simulink model "SimpleECU"  (R2024b)
settings: configuration reference "EngFixed10ms" (kept outside this file)
undefined symbols (not defined in the file): CtrlEcuRevLim
settings Model: DataDictionary=VirtualDynoTemplate.sldd  ModifiedByFormat=The MathWorks, Inc.  Creator=The MathWorks, Inc.  LastModifiedBy=The MathWorks, Inc.
settings ConfigSetRef: SourceName=EngFixed10ms

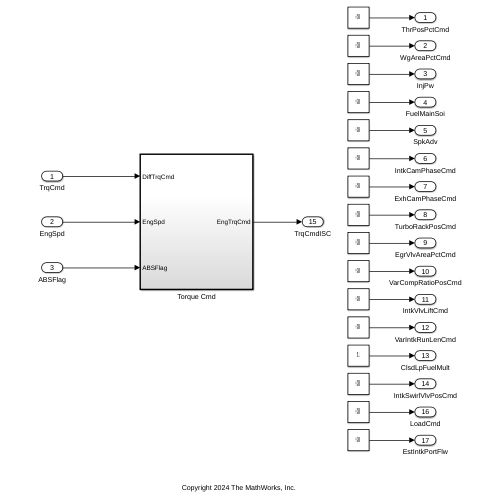
[thumbnail: Simulink's stored preview of the top-level diagram]
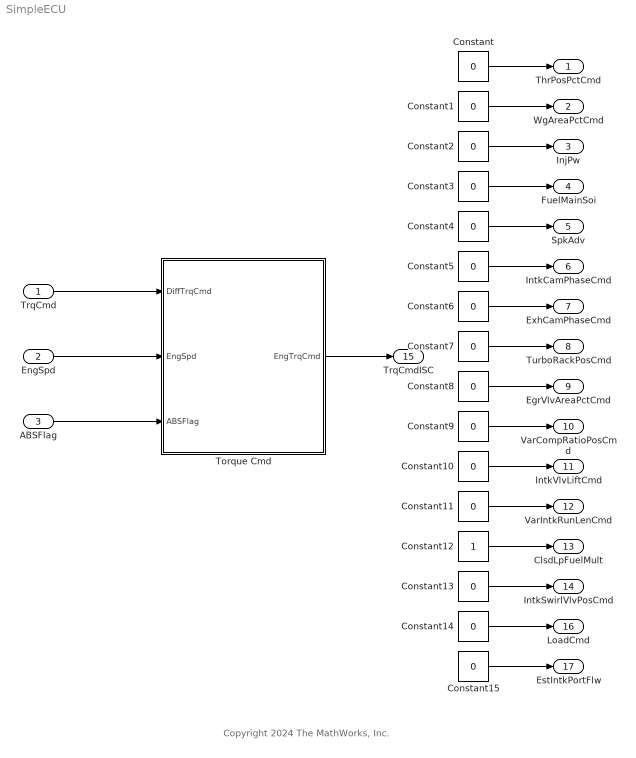
== system SimpleECU ==
  note: Copyright 2024 The MathWorks, Inc.
  TrqCmd : Inport
  EngSpd : Inport  Port=2
  ABSFlag : Inport  Port=3  OutDataTypeStr=boolean
  Constant{,1..11,13..15} (15 alike) : Constant  Value=0  SampleTime=-1
  Constant12 : Constant  SampleTime=-1
  Torque Cmd : Subsystem  TreatAsAtomicUnit=on  SystemSampleTime=.01
  ThrPosPctCmd : Outport  VectorParamsAs1DForOutWhenUnconnected=off
  WgAreaPctCmd : Outport  Port=2  VectorParamsAs1DForOutWhenUnconnected=off
  InjPw : Outport  Port=3  SampleTime=0.01  VectorParamsAs1DForOutWhenUnconnected=off
  FuelMainSoi : Outport  Port=4  Unit=deg  VectorParamsAs1DForOutWhenUnconnected=off
  SpkAdv : Outport  Port=5  VectorParamsAs1DForOutWhenUnconnected=off
  IntkCamPhaseCmd : Outport  Port=6  VectorParamsAs1DForOutWhenUnconnected=off
  ExhCamPhaseCmd : Outport  Port=7  VectorParamsAs1DForOutWhenUnconnected=off
  TurboRackPosCmd : Outport  Port=8  Unit=1  VectorParamsAs1DForOutWhenUnconnected=off
  EgrVlvAreaPctCmd : Outport  Port=9  Unit=%  VectorParamsAs1DForOutWhenUnconnected=off
  VarCompRatioPosCmd : Outport  Port=10  VectorParamsAs1DForOutWhenUnconnected=off
  IntkVlvLiftCmd : Outport  Port=11  VectorParamsAs1DForOutWhenUnconnected=off
  VarIntkRunLenCmd : Outport  Port=12  VectorParamsAs1DForOutWhenUnconnected=off
  ClsdLpFuelMult : Outport  Port=13  SampleTime=0.01  VectorParamsAs1DForOutWhenUnconnected=off
  IntkSwirlVlvPosCmd : Outport  Port=14  VectorParamsAs1DForOutWhenUnconnected=off
  TrqCmdISC : Outport  Port=15  VectorParamsAs1DForOutWhenUnconnected=off
  LoadCmd : Outport  Port=16  VectorParamsAs1DForOutWhenUnconnected=off
  EstIntkPortFlw : Outport  Port=17  VectorParamsAs1DForOutWhenUnconnected=off
  wires:
  ABSFlag/1 -> Torque Cmd/3(ABSFlag)
  Constant6/1 -> ExhCamPhaseCmd/1
  Constant9/1 -> VarCompRatioPosCmd/1
  Constant2/1 -> InjPw/1
  Constant1/1 -> WgAreaPctCmd/1
  Constant7/1 -> TurboRackPosCmd/1
  Constant14/1 -> LoadCmd/1
  Constant10/1 -> IntkVlvLiftCmd/1
  Constant8/1 -> EgrVlvAreaPctCmd/1
  Constant15/1 -> EstIntkPortFlw/1
  Torque Cmd/1(EngTrqCmd) -> TrqCmdISC/1
  Constant11/1 -> VarIntkRunLenCmd/1
  TrqCmd/1 -> Torque Cmd/1(DiffTrqCmd)
  Constant4/1 -> SpkAdv/1
  Constant3/1 -> FuelMainSoi/1
  Constant5/1 -> IntkCamPhaseCmd/1
  Constant/1 -> ThrPosPctCmd/1
  Constant13/1 -> IntkSwirlVlvPosCmd/1
  Constant12/1 -> ClsdLpFuelMult/1
  EngSpd/1 -> Torque Cmd/2(EngSpd)

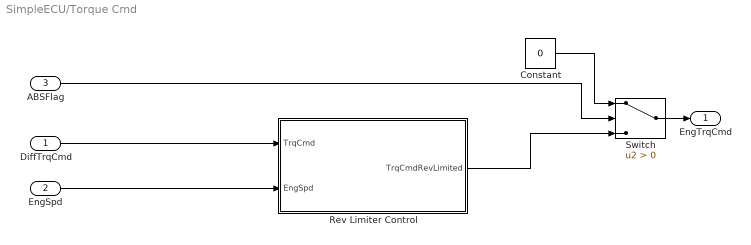
== system SimpleECU/Torque Cmd ==
  DiffTrqCmd : Inport
  EngSpd : Inport  Port=2  Unit=rpm
  ABSFlag : Inport  Port=3
  Constant : Constant  Value=0  SampleTime=-1
  Rev Limiter Control : Subsystem
  Switch : Switch  Criteria=u2 > Threshold  ZeroCross=off  SaturateOnIntegerOverflow=off  InputSameDT=off
  EngTrqCmd : Outport
  wires:
  DiffTrqCmd/1 -> Rev Limiter Control/1(TrqCmd)
  EngSpd/1 -> Rev Limiter Control/2(EngSpd)
  Rev Limiter Control/1(TrqCmdRevLimited) -> Switch/3
  Switch/1 -> EngTrqCmd/1
  Constant/1 -> Switch/1
  ABSFlag/1 -> Switch/2

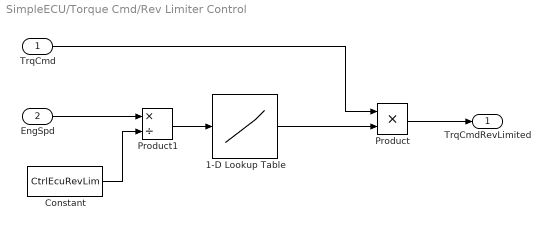
== system SimpleECU/Torque Cmd/Rev Limiter Control ==
  TrqCmd : Inport
  EngSpd : Inport  Port=2
  1-D Lookup Table : Lookup_n-D  NumberOfTableDimensions=1  BreakpointsForDimension1=[1 1.01]  Table=[1 0]  ExtrapMethod=Clip  InternalRulePriority=Speed  RndMeth=Simplest
  Constant : Constant  Value=CtrlEcuRevLim  SampleTime=-1
  Product : Product
  Product1 : Product  Inputs=*/
  TrqCmdRevLimited : Outport  VectorParamsAs1DForOutWhenUnconnected=off
  wires:
  EngSpd/1 -> Product1/1
  Product/1 -> TrqCmdRevLimited/1
  1-D Lookup Table/1 -> Product/2
  TrqCmd/1 -> Product/1
  Constant/1 -> Product1/2
  Product1/1 -> 1-D Lookup Table/1
